simulink model "TetheredUAV_Model"  (R2018a)
settings: Solver=VariableStepAuto  StartTime=0.0  StopTime=200  RelTol=1e-3
undefined symbols (not defined in the file): Discrete, Time, X, Y, Z
libraries: sm_lib x20, simulink x18, nesl_utility x16, commchan3 x5, sharedtransform x1, ctrlSharedLib x1
(part 2 of 2)

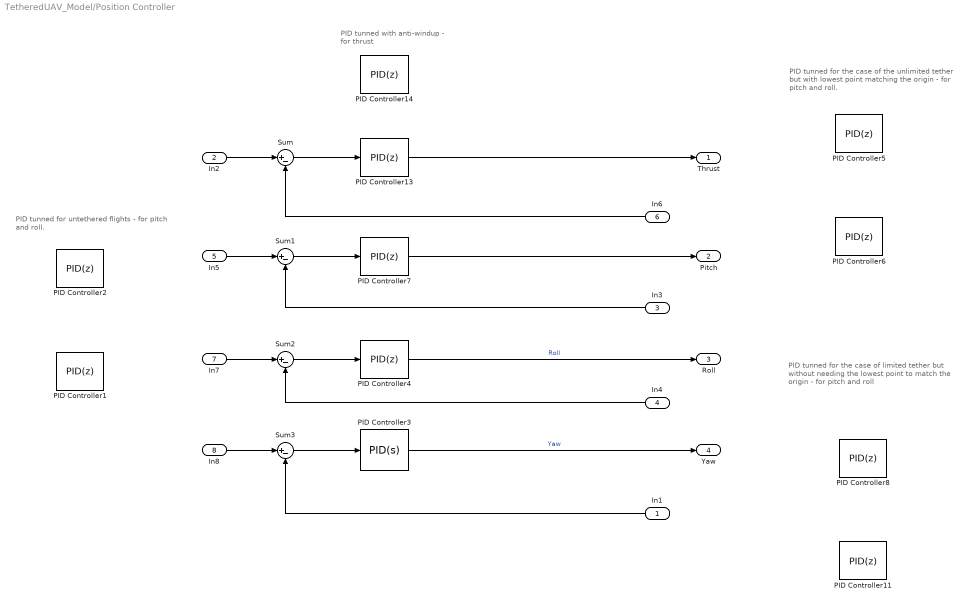
== system TetheredUAV_Model/Position Controller ==
  note: PID tunned with
      | anti-windup - for thrust
  note: PID tunned for the case of the
      | unlimited tether but with lowest
      | point matching the origin - for pitch
      | and roll.
  note: PID tunned for untethered flights -
      | for pitch and roll.
  note: PID tunned for the case of limited
      | tether but without needing the
      | lowest point to match the origin - for
      | pitch and roll
  In1 : Inport
  In2 : Inport  Port=2
  In3 : Inport  Port=3
  In4 : Inport  Port=4
  In5 : Inport  Port=5
  In6 : Inport  Port=6
  In7 : Inport  Port=7
  In8 : Inport  Port=8
  PID Controller1 : simulink/Continuous/PID Controller  Controller=PID  TimeDomain=Discrete-time  SampleTime=0.01  IntegratorMethod=Forward Euler  FilterMethod=Forward Euler  Form=Parallel  UseFilter=off  ControllerParametersSource=internal  P=-0.160436022246273  I=0  D=0  N=44.4052744202431  InitialConditionSource=internal  InitialConditionForIntegrator=0  InitialConditionForFilter=0  ExternalReset=none  LimitOutput=on  UpperSaturationLimit=10  LowerSaturationLimit=-10  LinearizeAsGain=on  AntiWindupMode=none  Kb=1  TrackingMode=off  Kt=1  PParamMin=[]  PParamMax=[]  IParamMin=[]  IParamMax=[]  DParamMin=[]  DParamMax=[]  NParamMin=[]  NParamMax=[]  KbParamMin=[]  KbParamMax=[]  KtParamMin=[]  KtParamMax=[]  POutMin=[]  POutMax=[]  IOutMin=[]  IOutMax=[]  DOutMin=[]  DOutMax=[]  NOutMin=[]  NOutMax=[]  KbOutMin=[]  KbOutMax=[]  KtOutMin=[]  KtOutMax=[]  IntegratorOutMin=[]  IntegratorOutMax=[]  FilterOutMin=[]  FilterOutMax=[]  SumOutMin=[]  SumOutMax=[]  SumI1OutMin=[]  SumI1OutMax=[]  SumI2OutMin=[]  SumI2OutMax=[]  SumI3OutMin=[]  SumI3OutMax=[]  SumDOutMin=[]  SumDOutMax=[]  SaturationOutMin=[]  SaturationOutMax=[]  IntegratorContinuousStateAttributes=''  IntegratorStateMustResolveToSignalObject=off  IntegratorRTWStateStorageClass=Auto  FilterContinuousStateAttributes=''  FilterStateMustResolveToSignalObject=off  FilterRTWStateStorageClass=Auto  DifferentiatorICPrevScaledInput=0  DifferentiatorOutMin=[]  DifferentiatorOutMax=[]  FilterDiffOutCoefMin=[]  FilterDiffOutCoefMax=[]  SumDenOutMin=[]  SumDenOutMax=[]  SumNumOutMin=[]  SumNumOutMax=[]  ReciprocalOutMin=[]  ReciprocalOutMax=[]  DivideOutMin=[]  DivideOutMax=[]  TunerSelectOption=Transfer Function Based (PID Tuner App)
  PID Controller11 : simulink/Continuous/PID Controller  Controller=PID  TimeDomain=Discrete-time  SampleTime=0.01  IntegratorMethod=Forward Euler  FilterMethod=Forward Euler  Form=Parallel  UseFilter=off  ControllerParametersSource=internal  P=-0.1  I=-0.2  D=-15  N=44.4052744202431  InitialConditionSource=internal  InitialConditionForIntegrator=0  InitialConditionForFilter=0  ExternalReset=none  LimitOutput=on  UpperSaturationLimit=10  LowerSaturationLimit=-10  LinearizeAsGain=on  AntiWindupMode=none  Kb=1  TrackingMode=off  Kt=1  PParamMin=[]  PParamMax=[]  IParamMin=[]  IParamMax=[]  DParamMin=[]  DParamMax=[]  NParamMin=[]  NParamMax=[]  KbParamMin=[]  KbParamMax=[]  KtParamMin=[]  KtParamMax=[]  POutMin=[]  POutMax=[]  IOutMin=[]  IOutMax=[]  DOutMin=[]  DOutMax=[]  NOutMin=[]  NOutMax=[]  KbOutMin=[]  KbOutMax=[]  KtOutMin=[]  KtOutMax=[]  IntegratorOutMin=[]  IntegratorOutMax=[]  FilterOutMin=[]  FilterOutMax=[]  SumOutMin=[]  SumOutMax=[]  SumI1OutMin=[]  SumI1OutMax=[]  SumI2OutMin=[]  SumI2OutMax=[]  SumI3OutMin=[]  SumI3OutMax=[]  SumDOutMin=[]  SumDOutMax=[]  SaturationOutMin=[]  SaturationOutMax=[]  IntegratorContinuousStateAttributes=''  IntegratorStateMustResolveToSignalObject=off  IntegratorRTWStateStorageClass=Auto  FilterContinuousStateAttributes=''  FilterStateMustResolveToSignalObject=off  FilterRTWStateStorageClass=Auto  DifferentiatorICPrevScaledInput=0  DifferentiatorOutMin=[]  DifferentiatorOutMax=[]  FilterDiffOutCoefMin=[]  FilterDiffOutCoefMax=[]  SumDenOutMin=[]  SumDenOutMax=[]  SumNumOutMin=[]  SumNumOutMax=[]  ReciprocalOutMin=[]  ReciprocalOutMax=[]  DivideOutMin=[]  DivideOutMax=[]  TunerSelectOption=Transfer Function Based (PID Tuner App)
  PID Controller13 : simulink/Continuous/PID Controller  Controller=PID  TimeDomain=Discrete-time  SampleTime=0.01  IntegratorMethod=Forward Euler  FilterMethod=Forward Euler  Form=Parallel  UseFilter=off  ControllerParametersSource=internal  P=140000  I=7000  D=1000000  N=1  InitialConditionSource=internal  InitialConditionForIntegrator=0  InitialConditionForFilter=0  ExternalReset=none  LimitOutput=on  UpperSaturationLimit=240000  LowerSaturationLimit=40000  LinearizeAsGain=on  AntiWindupMode=none  Kb=1  TrackingMode=off  Kt=1  PParamMin=[]  PParamMax=[]  IParamMin=[]  IParamMax=[]  DParamMin=[]  DParamMax=[]  NParamMin=[]  NParamMax=[]  KbParamMin=[]  KbParamMax=[]  KtParamMin=[]  KtParamMax=[]  POutMin=[]  POutMax=[]  IOutMin=[]  IOutMax=[]  DOutMin=[]  DOutMax=[]  NOutMin=[]  NOutMax=[]  KbOutMin=[]  KbOutMax=[]  KtOutMin=[]  KtOutMax=[]  IntegratorOutMin=[]  IntegratorOutMax=[]  FilterOutMin=[]  FilterOutMax=[]  SumOutMin=[]  SumOutMax=[]  SumI1OutMin=[]  SumI1OutMax=[]  SumI2OutMin=[]  SumI2OutMax=[]  SumI3OutMin=[]  SumI3OutMax=[]  SumDOutMin=[]  SumDOutMax=[]  SaturationOutMin=[]  SaturationOutMax=[]  IntegratorContinuousStateAttributes=''  IntegratorStateMustResolveToSignalObject=off  IntegratorRTWStateStorageClass=Auto  FilterContinuousStateAttributes=''  FilterStateMustResolveToSignalObject=off  FilterRTWStateStorageClass=Auto  DifferentiatorICPrevScaledInput=0  DifferentiatorOutMin=[]  DifferentiatorOutMax=[]  FilterDiffOutCoefMin=[]  FilterDiffOutCoefMax=[]  SumDenOutMin=[]  SumDenOutMax=[]  SumNumOutMin=[]  SumNumOutMax=[]  ReciprocalOutMin=[]  ReciprocalOutMax=[]  DivideOutMin=[]  DivideOutMax=[]  TunerSelectOption=Transfer Function Based (PID Tuner App)
  PID Controller14 : simulink/Continuous/PID Controller  Controller=PID  TimeDomain=Discrete-time  SampleTime=0.01  IntegratorMethod=Forward Euler  FilterMethod=Forward Euler  Form=Parallel  UseFilter=off  ControllerParametersSource=internal  P=140000  I=10000  D=1000000  N=1  InitialConditionSource=internal  InitialConditionForIntegrator=0  InitialConditionForFilter=0  ExternalReset=none  LimitOutput=on  UpperSaturationLimit=240000  LowerSaturationLimit=40000  LinearizeAsGain=on  AntiWindupMode=back-calculation  Kb=1  TrackingMode=off  Kt=1  PParamMin=[]  PParamMax=[]  IParamMin=[]  IParamMax=[]  DParamMin=[]  DParamMax=[]  NParamMin=[]  NParamMax=[]  KbParamMin=[]  KbParamMax=[]  KtParamMin=[]  KtParamMax=[]  POutMin=[]  POutMax=[]  IOutMin=[]  IOutMax=[]  DOutMin=[]  DOutMax=[]  NOutMin=[]  NOutMax=[]  KbOutMin=[]  KbOutMax=[]  KtOutMin=[]  KtOutMax=[]  IntegratorOutMin=[]  IntegratorOutMax=[]  FilterOutMin=[]  FilterOutMax=[]  SumOutMin=[]  SumOutMax=[]  SumI1OutMin=[]  SumI1OutMax=[]  SumI2OutMin=[]  SumI2OutMax=[]  SumI3OutMin=[]  SumI3OutMax=[]  SumDOutMin=[]  SumDOutMax=[]  SaturationOutMin=[]  SaturationOutMax=[]  IntegratorContinuousStateAttributes=''  IntegratorStateMustResolveToSignalObject=off  IntegratorRTWStateStorageClass=Auto  FilterContinuousStateAttributes=''  FilterStateMustResolveToSignalObject=off  FilterRTWStateStorageClass=Auto  DifferentiatorICPrevScaledInput=0  DifferentiatorOutMin=[]  DifferentiatorOutMax=[]  FilterDiffOutCoefMin=[]  FilterDiffOutCoefMax=[]  SumDenOutMin=[]  SumDenOutMax=[]  SumNumOutMin=[]  SumNumOutMax=[]  ReciprocalOutMin=[]  ReciprocalOutMax=[]  DivideOutMin=[]  DivideOutMax=[]  TunerSelectOption=Transfer Function Based (PID Tuner App)
  PID Controller2 : simulink/Continuous/PID Controller  Controller=PID  TimeDomain=Discrete-time  SampleTime=0.01  IntegratorMethod=Forward Euler  FilterMethod=Forward Euler  Form=Parallel  UseFilter=off  ControllerParametersSource=internal  P=0.160436022246273  I=0  D=0  N=44.4052744202431  InitialConditionSource=internal  InitialConditionForIntegrator=0  InitialConditionForFilter=0  ExternalReset=none  LimitOutput=on  UpperSaturationLimit=10  LowerSaturationLimit=-10  LinearizeAsGain=on  AntiWindupMode=none  Kb=1  TrackingMode=off  Kt=1  PParamMin=[]  PParamMax=[]  IParamMin=[]  IParamMax=[]  DParamMin=[]  DParamMax=[]  NParamMin=[]  NParamMax=[]  KbParamMin=[]  KbParamMax=[]  KtParamMin=[]  KtParamMax=[]  POutMin=[]  POutMax=[]  IOutMin=[]  IOutMax=[]  DOutMin=[]  DOutMax=[]  NOutMin=[]  NOutMax=[]  KbOutMin=[]  KbOutMax=[]  KtOutMin=[]  KtOutMax=[]  IntegratorOutMin=[]  IntegratorOutMax=[]  FilterOutMin=[]  FilterOutMax=[]  SumOutMin=[]  SumOutMax=[]  SumI1OutMin=[]  SumI1OutMax=[]  SumI2OutMin=[]  SumI2OutMax=[]  SumI3OutMin=[]  SumI3OutMax=[]  SumDOutMin=[]  SumDOutMax=[]  SaturationOutMin=[]  SaturationOutMax=[]  IntegratorContinuousStateAttributes=''  IntegratorStateMustResolveToSignalObject=off  IntegratorRTWStateStorageClass=Auto  FilterContinuousStateAttributes=''  FilterStateMustResolveToSignalObject=off  FilterRTWStateStorageClass=Auto  DifferentiatorICPrevScaledInput=0  DifferentiatorOutMin=[]  DifferentiatorOutMax=[]  FilterDiffOutCoefMin=[]  FilterDiffOutCoefMax=[]  SumDenOutMin=[]  SumDenOutMax=[]  SumNumOutMin=[]  SumNumOutMax=[]  ReciprocalOutMin=[]  ReciprocalOutMax=[]  DivideOutMin=[]  DivideOutMax=[]  TunerSelectOption=Transfer Function Based (PID Tuner App)
  PID Controller3 : simulink/Continuous/PID Controller  Controller=PID  TimeDomain=Continuous-time  SampleTime=-1  IntegratorMethod=Forward Euler  FilterMethod=Forward Euler  Form=Parallel  UseFilter=on  ControllerParametersSource=internal  P=0  I=0  D=0  N=5.45397025421619  InitialConditionSource=internal  InitialConditionForIntegrator=0  InitialConditionForFilter=0  ExternalReset=none  LimitOutput=off  UpperSaturationLimit=inf  LowerSaturationLimit=-inf  LinearizeAsGain=on  AntiWindupMode=none  Kb=1  TrackingMode=off  Kt=1  PParamMin=[]  PParamMax=[]  IParamMin=[]  IParamMax=[]  DParamMin=[]  DParamMax=[]  NParamMin=[]  NParamMax=[]  KbParamMin=[]  KbParamMax=[]  KtParamMin=[]  KtParamMax=[]  POutMin=[]  POutMax=[]  IOutMin=[]  IOutMax=[]  DOutMin=[]  DOutMax=[]  NOutMin=[]  NOutMax=[]  KbOutMin=[]  KbOutMax=[]  KtOutMin=[]  KtOutMax=[]  IntegratorOutMin=[]  IntegratorOutMax=[]  FilterOutMin=[]  FilterOutMax=[]  SumOutMin=[]  SumOutMax=[]  SumI1OutMin=[]  SumI1OutMax=[]  SumI2OutMin=[]  SumI2OutMax=[]  SumI3OutMin=[]  SumI3OutMax=[]  SumDOutMin=[]  SumDOutMax=[]  SaturationOutMin=[]  SaturationOutMax=[]  IntegratorContinuousStateAttributes=''  IntegratorStateMustResolveToSignalObject=off  IntegratorRTWStateStorageClass=Auto  FilterContinuousStateAttributes=''  FilterStateMustResolveToSignalObject=off  FilterRTWStateStorageClass=Auto  DifferentiatorICPrevScaledInput=0  DifferentiatorOutMin=[]  DifferentiatorOutMax=[]  FilterDiffOutCoefMin=[]  FilterDiffOutCoefMax=[]  SumDenOutMin=[]  SumDenOutMax=[]  SumNumOutMin=[]  SumNumOutMax=[]  ReciprocalOutMin=[]  ReciprocalOutMax=[]  DivideOutMin=[]  DivideOutMax=[]  TunerSelectOption=Transfer Function Based (PID Tuner App)
  PID Controller4 : simulink/Continuous/PID Controller  Controller=PID  TimeDomain=Discrete-time  SampleTime=0.01  IntegratorMethod=Forward Euler  FilterMethod=Forward Euler  Form=Parallel  UseFilter=off  ControllerParametersSource=internal  P=-0.1  I=-0.2  D=-15  N=44.4052744202431  InitialConditionSource=internal  InitialConditionForIntegrator=0  InitialConditionForFilter=0  ExternalReset=none  LimitOutput=on  UpperSaturationLimit=10  LowerSaturationLimit=-10  LinearizeAsGain=on  AntiWindupMode=none  Kb=1  TrackingMode=off  Kt=1  PParamMin=[]  PParamMax=[]  IParamMin=[]  IParamMax=[]  DParamMin=[]  DParamMax=[]  NParamMin=[]  NParamMax=[]  KbParamMin=[]  KbParamMax=[]  KtParamMin=[]  KtParamMax=[]  POutMin=[]  POutMax=[]  IOutMin=[]  IOutMax=[]  DOutMin=[]  DOutMax=[]  NOutMin=[]  NOutMax=[]  KbOutMin=[]  KbOutMax=[]  KtOutMin=[]  KtOutMax=[]  IntegratorOutMin=[]  IntegratorOutMax=[]  FilterOutMin=[]  FilterOutMax=[]  SumOutMin=[]  SumOutMax=[]  SumI1OutMin=[]  SumI1OutMax=[]  SumI2OutMin=[]  SumI2OutMax=[]  SumI3OutMin=[]  SumI3OutMax=[]  SumDOutMin=[]  SumDOutMax=[]  SaturationOutMin=[]  SaturationOutMax=[]  IntegratorContinuousStateAttributes=''  IntegratorStateMustResolveToSignalObject=off  IntegratorRTWStateStorageClass=Auto  FilterContinuousStateAttributes=''  FilterStateMustResolveToSignalObject=off  FilterRTWStateStorageClass=Auto  DifferentiatorICPrevScaledInput=0  DifferentiatorOutMin=[]  DifferentiatorOutMax=[]  FilterDiffOutCoefMin=[]  FilterDiffOutCoefMax=[]  SumDenOutMin=[]  SumDenOutMax=[]  SumNumOutMin=[]  SumNumOutMax=[]  ReciprocalOutMin=[]  ReciprocalOutMax=[]  DivideOutMin=[]  DivideOutMax=[]  TunerSelectOption=Transfer Function Based (PID Tuner App)
  PID Controller5 : simulink/Continuous/PID Controller  Controller=PID  TimeDomain=Discrete-time  SampleTime=0.01  IntegratorMethod=Forward Euler  FilterMethod=Forward Euler  Form=Parallel  UseFilter=off  ControllerParametersSource=internal  P=0.4  I=0.4  D=2  N=44.4052744202431  InitialConditionSource=internal  InitialConditionForIntegrator=0  InitialConditionForFilter=0  ExternalReset=none  LimitOutput=on  UpperSaturationLimit=10  LowerSaturationLimit=-10  LinearizeAsGain=on  AntiWindupMode=none  Kb=1  TrackingMode=off  Kt=1  PParamMin=[]  PParamMax=[]  IParamMin=[]  IParamMax=[]  DParamMin=[]  DParamMax=[]  NParamMin=[]  NParamMax=[]  KbParamMin=[]  KbParamMax=[]  KtParamMin=[]  KtParamMax=[]  POutMin=[]  POutMax=[]  IOutMin=[]  IOutMax=[]  DOutMin=[]  DOutMax=[]  NOutMin=[]  NOutMax=[]  KbOutMin=[]  KbOutMax=[]  KtOutMin=[]  KtOutMax=[]  IntegratorOutMin=[]  IntegratorOutMax=[]  FilterOutMin=[]  FilterOutMax=[]  SumOutMin=[]  SumOutMax=[]  SumI1OutMin=[]  SumI1OutMax=[]  SumI2OutMin=[]  SumI2OutMax=[]  SumI3OutMin=[]  SumI3OutMax=[]  SumDOutMin=[]  SumDOutMax=[]  SaturationOutMin=[]  SaturationOutMax=[]  IntegratorContinuousStateAttributes=''  IntegratorStateMustResolveToSignalObject=off  IntegratorRTWStateStorageClass=Auto  FilterContinuousStateAttributes=''  FilterStateMustResolveToSignalObject=off  FilterRTWStateStorageClass=Auto  DifferentiatorICPrevScaledInput=0  DifferentiatorOutMin=[]  DifferentiatorOutMax=[]  FilterDiffOutCoefMin=[]  FilterDiffOutCoefMax=[]  SumDenOutMin=[]  SumDenOutMax=[]  SumNumOutMin=[]  SumNumOutMax=[]  ReciprocalOutMin=[]  ReciprocalOutMax=[]  DivideOutMin=[]  DivideOutMax=[]  TunerSelectOption=Transfer Function Based (PID Tuner App)
  PID Controller6 : simulink/Continuous/PID Controller  Controller=PID  TimeDomain=Discrete-time  SampleTime=0.01  IntegratorMethod=Forward Euler  FilterMethod=Forward Euler  Form=Parallel  UseFilter=off  ControllerParametersSource=internal  P=-0.4  I=-0.4  D=-2  N=44.4052744202431  InitialConditionSource=internal  InitialConditionForIntegrator=0  InitialConditionForFilter=0  ExternalReset=none  LimitOutput=on  UpperSaturationLimit=10  LowerSaturationLimit=-10  LinearizeAsGain=on  AntiWindupMode=none  Kb=1  TrackingMode=off  Kt=1  PParamMin=[]  PParamMax=[]  IParamMin=[]  IParamMax=[]  DParamMin=[]  DParamMax=[]  NParamMin=[]  NParamMax=[]  KbParamMin=[]  KbParamMax=[]  KtParamMin=[]  KtParamMax=[]  POutMin=[]  POutMax=[]  IOutMin=[]  IOutMax=[]  DOutMin=[]  DOutMax=[]  NOutMin=[]  NOutMax=[]  KbOutMin=[]  KbOutMax=[]  KtOutMin=[]  KtOutMax=[]  IntegratorOutMin=[]  IntegratorOutMax=[]  FilterOutMin=[]  FilterOutMax=[]  SumOutMin=[]  SumOutMax=[]  SumI1OutMin=[]  SumI1OutMax=[]  SumI2OutMin=[]  SumI2OutMax=[]  SumI3OutMin=[]  SumI3OutMax=[]  SumDOutMin=[]  SumDOutMax=[]  SaturationOutMin=[]  SaturationOutMax=[]  IntegratorContinuousStateAttributes=''  IntegratorStateMustResolveToSignalObject=off  IntegratorRTWStateStorageClass=Auto  FilterContinuousStateAttributes=''  FilterStateMustResolveToSignalObject=off  FilterRTWStateStorageClass=Auto  DifferentiatorICPrevScaledInput=0  DifferentiatorOutMin=[]  DifferentiatorOutMax=[]  FilterDiffOutCoefMin=[]  FilterDiffOutCoefMax=[]  SumDenOutMin=[]  SumDenOutMax=[]  SumNumOutMin=[]  SumNumOutMax=[]  ReciprocalOutMin=[]  ReciprocalOutMax=[]  DivideOutMin=[]  DivideOutMax=[]  TunerSelectOption=Transfer Function Based (PID Tuner App)
  PID Controller7 : simulink/Continuous/PID Controller  Controller=PID  TimeDomain=Discrete-time  SampleTime=0.01  IntegratorMethod=Forward Euler  FilterMethod=Forward Euler  Form=Parallel  UseFilter=off  ControllerParametersSource=internal  P=0.1  I=0.2  D=15  N=44.4052744202431  InitialConditionSource=internal  InitialConditionForIntegrator=0  InitialConditionForFilter=0  ExternalReset=none  LimitOutput=on  UpperSaturationLimit=10  LowerSaturationLimit=-10  LinearizeAsGain=on  AntiWindupMode=none  Kb=1  TrackingMode=off  Kt=1  PParamMin=[]  PParamMax=[]  IParamMin=[]  IParamMax=[]  DParamMin=[]  DParamMax=[]  NParamMin=[]  NParamMax=[]  KbParamMin=[]  KbParamMax=[]  KtParamMin=[]  KtParamMax=[]  POutMin=[]  POutMax=[]  IOutMin=[]  IOutMax=[]  DOutMin=[]  DOutMax=[]  NOutMin=[]  NOutMax=[]  KbOutMin=[]  KbOutMax=[]  KtOutMin=[]  KtOutMax=[]  IntegratorOutMin=[]  IntegratorOutMax=[]  FilterOutMin=[]  FilterOutMax=[]  SumOutMin=[]  SumOutMax=[]  SumI1OutMin=[]  SumI1OutMax=[]  SumI2OutMin=[]  SumI2OutMax=[]  SumI3OutMin=[]  SumI3OutMax=[]  SumDOutMin=[]  SumDOutMax=[]  SaturationOutMin=[]  SaturationOutMax=[]  IntegratorContinuousStateAttributes=''  IntegratorStateMustResolveToSignalObject=off  IntegratorRTWStateStorageClass=Auto  FilterContinuousStateAttributes=''  FilterStateMustResolveToSignalObject=off  FilterRTWStateStorageClass=Auto  DifferentiatorICPrevScaledInput=0  DifferentiatorOutMin=[]  DifferentiatorOutMax=[]  FilterDiffOutCoefMin=[]  FilterDiffOutCoefMax=[]  SumDenOutMin=[]  SumDenOutMax=[]  SumNumOutMin=[]  SumNumOutMax=[]  ReciprocalOutMin=[]  ReciprocalOutMax=[]  DivideOutMin=[]  DivideOutMax=[]  TunerSelectOption=Transfer Function Based (PID Tuner App)
  PID Controller8 : simulink/Continuous/PID Controller  Controller=PID  TimeDomain=Discrete-time  SampleTime=0.01  IntegratorMethod=Forward Euler  FilterMethod=Forward Euler  Form=Parallel  UseFilter=off  ControllerParametersSource=internal  P=0.1  I=0.2  D=15  N=44.4052744202431  InitialConditionSource=internal  InitialConditionForIntegrator=0  InitialConditionForFilter=0  ExternalReset=none  LimitOutput=on  UpperSaturationLimit=10  LowerSaturationLimit=-10  LinearizeAsGain=on  AntiWindupMode=none  Kb=1  TrackingMode=off  Kt=1  PParamMin=[]  PParamMax=[]  IParamMin=[]  IParamMax=[]  DParamMin=[]  DParamMax=[]  NParamMin=[]  NParamMax=[]  KbParamMin=[]  KbParamMax=[]  KtParamMin=[]  KtParamMax=[]  POutMin=[]  POutMax=[]  IOutMin=[]  IOutMax=[]  DOutMin=[]  DOutMax=[]  NOutMin=[]  NOutMax=[]  KbOutMin=[]  KbOutMax=[]  KtOutMin=[]  KtOutMax=[]  IntegratorOutMin=[]  IntegratorOutMax=[]  FilterOutMin=[]  FilterOutMax=[]  SumOutMin=[]  SumOutMax=[]  SumI1OutMin=[]  SumI1OutMax=[]  SumI2OutMin=[]  SumI2OutMax=[]  SumI3OutMin=[]  SumI3OutMax=[]  SumDOutMin=[]  SumDOutMax=[]  SaturationOutMin=[]  SaturationOutMax=[]  IntegratorContinuousStateAttributes=''  IntegratorStateMustResolveToSignalObject=off  IntegratorRTWStateStorageClass=Auto  FilterContinuousStateAttributes=''  FilterStateMustResolveToSignalObject=off  FilterRTWStateStorageClass=Auto  DifferentiatorICPrevScaledInput=0  DifferentiatorOutMin=[]  DifferentiatorOutMax=[]  FilterDiffOutCoefMin=[]  FilterDiffOutCoefMax=[]  SumDenOutMin=[]  SumDenOutMax=[]  SumNumOutMin=[]  SumNumOutMax=[]  ReciprocalOutMin=[]  ReciprocalOutMax=[]  DivideOutMin=[]  DivideOutMax=[]  TunerSelectOption=Transfer Function Based (PID Tuner App)
  Sum{,1..3} (4 alike) : Sum  Inputs=|+-
  Thrust : Outport
  Pitch : Outport  Port=2
  Roll : Outport  Port=3
  Yaw : Outport  Port=4
  wires:
  Sum3/1 -> PID Controller3/1
  In1/1 -> Sum3/2
  PID Controller4/1 -> Roll/1  "Roll"
  In8/1 -> Sum3/1
  In2/1 -> Sum/1
  Sum2/1 -> PID Controller4/1
  In6/1 -> Sum/2
  PID Controller3/1 -> Yaw/1  "Yaw"
  In4/1 -> Sum2/2
  PID Controller7/1 -> Pitch/1
  Sum1/1 -> PID Controller7/1
  Sum/1 -> PID Controller13/1
  PID Controller13/1 -> Thrust/1
  In3/1 -> Sum1/2
  In5/1 -> Sum1/1
  In7/1 -> Sum2/1

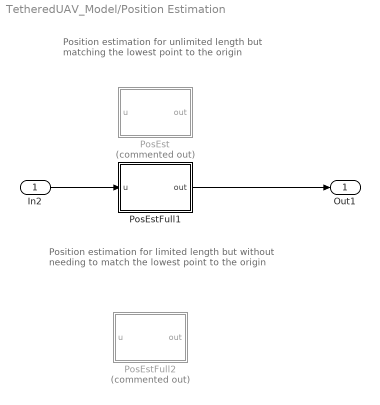
== system TetheredUAV_Model/Position Estimation ==
  note: Position estimation for limited length
      | but without needing to match the
      | lowest point to the origin
  note: Position estimation for unlimited
      | length but matching the lowest point
      | to the origin
  In2 : Inport
  PosEst : MATLAB Function  Commented=on  TreatAsAtomicUnit=on
  PosEstFull1 : MATLAB Function  TreatAsAtomicUnit=on
  PosEstFull2 : MATLAB Function  Commented=on  TreatAsAtomicUnit=on
  Out1 : Outport
  wires:
  PosEstFull1/1(out) -> Out1/1
  In2/1 -> PosEstFull1/1(u)

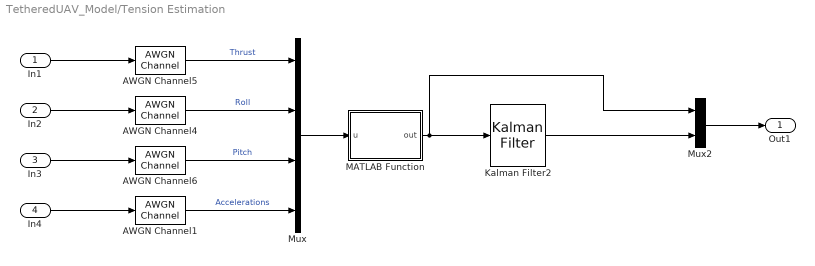
== system TetheredUAV_Model/Tension Estimation ==
  In1 : Inport
  In2 : Inport  Port=2
  In3 : Inport  Port=3
  In4 : Inport  Port=4
  AWGN Channel1 : commchan3/AWGN Channel  InputProcessing=Columns as channels (frame based)  seed=67  noiseMode="Signal to noise ratio  (SNR)"  EbNodB=10  EsNodB=10  SNRdB=30  bitsPerSym=1  Ps=1  Tsym=1  variance=1
  AWGN Channel4 : commchan3/AWGN Channel  InputProcessing=Columns as channels (frame based)  seed=67  noiseMode="Signal to noise ratio  (SNR)"  EbNodB=10  EsNodB=10  SNRdB=40  bitsPerSym=1  Ps=1  Tsym=1  variance=1
  AWGN Channel5 : commchan3/AWGN Channel  InputProcessing=Columns as channels (frame based)  seed=67  noiseMode="Signal to noise ratio  (SNR)"  EbNodB=10  EsNodB=10  SNRdB=40  bitsPerSym=1  Ps=1  Tsym=1  variance=1
  AWGN Channel6 : commchan3/AWGN Channel  InputProcessing=Columns as channels (frame based)  seed=67  noiseMode="Signal to noise ratio  (SNR)"  EbNodB=10  EsNodB=10  SNRdB=40  bitsPerSym=1  Ps=1  Tsym=1  variance=1
  Kalman Filter2 : ctrlSharedLib/Kalman Filter  TimeDomain=Discrete-Time  UseCurrentEstimator=on  ModelSource=Individual A, B, C, D matrices  ModelSourceVariable=ss(0.95,1,1,0,1)  A=eye(3)  B=0  C=eye(3)  D=0  NumberOfStates=1  NumberOfInputs=1  NumberOfOutputs=1  InitialEstimateSource=Dialog  X0=0  P0=10  UseK=off  UseGH=off  NumberOfProcessNoiseInputs=1  G=1  TimeInvariantG=on  H=0  TimeInvariantH=on  Q=diag([1 1 1])  TimeInvariantQ=on  R=100000*eye(3)  TimeInvariantR=on  N=0  TimeInvariantN=on  AddInputPort=off  AddEnablePort=off  OutputEstimatedY=off  OutputP=off  Ts=-1
      settings: SourceProductBaseCode=CT
  MATLAB Function : MATLAB Function  TreatAsAtomicUnit=on
  Mux : Mux
  Mux2 : Mux  Inputs=2
  Out1 : Outport
  wires:
  Mux/1 -> MATLAB Function/1(u)
  Mux2/1 -> Out1/1
  MATLAB Function/1(out) -> Kalman Filter2/1, Mux2/1
  Kalman Filter2/1 -> Mux2/2
  In3/1 -> AWGN Channel6/1
  In2/1 -> AWGN Channel4/1
  In4/1 -> AWGN Channel1/1
  In1/1 -> AWGN Channel5/1
  AWGN Channel4/1 -> Mux/2  "Roll"
  AWGN Channel6/1 -> Mux/3  "Pitch"
  AWGN Channel1/1 -> Mux/4  "Accelerations"
  AWGN Channel5/1 -> Mux/1  "Thrust"

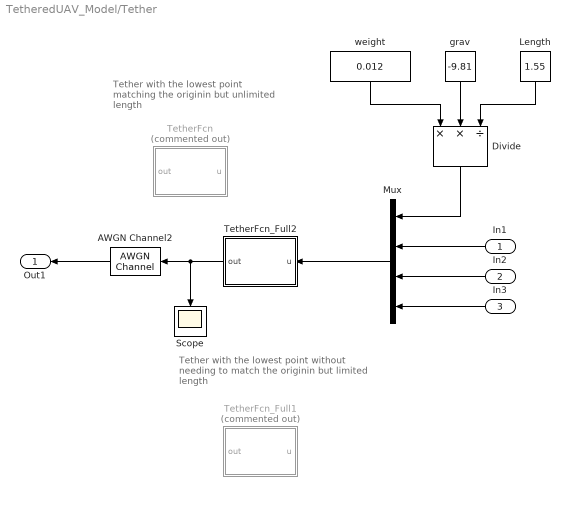
== system TetheredUAV_Model/Tether ==
  note: Tether with the lowest point
      | without needing to match the
      | originin but limited length
  note: Tether with the lowest point
      | matching the originin but
      | unlimited length
  In1 : Inport
  In2 : Inport  Port=2
  In3 : Inport  Port=3
  AWGN Channel2 : commchan3/AWGN Channel  InputProcessing=Columns as channels (frame based)  seed=67  noiseMode="Signal to noise ratio  (SNR)"  EbNodB=10  EsNodB=10  SNRdB=70  bitsPerSym=1  Ps=1  Tsym=1  variance=1
  Divide : Product  Inputs=**/
  Length : Constant  Value=1.55
  Mux : Mux
  Scope : Scope
  TetherFcn : MATLAB Function  Commented=on  TreatAsAtomicUnit=on
  TetherFcn_Full1 : MATLAB Function  Commented=on  TreatAsAtomicUnit=on
  TetherFcn_Full2 : MATLAB Function  TreatAsAtomicUnit=on
  grav : Constant  Value=-9.81
  weight : Constant  Value=0.012
  Out1 : Outport
  wires:
  TetherFcn_Full2/1(out) -> AWGN Channel2/1, Scope/1
  weight/1 -> Divide/1
  Length/1 -> Divide/3
  Divide/1 -> Mux/1
  In1/1 -> Mux/2
  In2/1 -> Mux/3
  In3/1 -> Mux/4
  Mux/1 -> TetherFcn_Full2/1(u)
  grav/1 -> Divide/2
  AWGN Channel2/1 -> Out1/1

== matlab function TetheredUAV_Model/Position Estimation/PosEstFull2 ==
  data: u input; out output
function out = fcn(u)
w=0.012/1.55*9.81;
s_tot=1.55;
% ---- Before Kalman - Raw observations
Tx=-u(4);
Ty=-u(5);
Tz=-u(6);
zi=0.754;
ri=0;

%Obtain the "a" and "s" parameters from the tension
T0=sqrt(Tx^2+Ty^2);
a=T0/w;
s=Tz/w;

%Obtain the r0, r(radial distance), C and z(altitude)
r0=a*asinh((s_tot-s)/a);
r=r0+a*asinh(s/a);
C=zi-a*cosh((ri-r0)/a);
z=a*cosh((r-r0)/a)+C;

%Decomposition of the r
teta=atan2(Ty,Tx);
y=r*sin(teta);
x=r*cos(teta);

out = [x,y,z];

== matlab function TetheredUAV_Model/Motor Controller/MATLAB Function1 ==
  data: u input; y output
function y = fcn(u)
f=u(1);
t1=u(2);
t2=u(3);
t3=u(4);

d=sqrt(2)/2*(0.5-0.025);
c=1;

vec=[f,t1,t2,t3]';
Matrix=[1,1,1,1;0,d,0,-d;-d,0,d,0;-c,c,-c,c];

y=(Matrix)\vec;
y=2.130925*10^(-11)*y.^2+1.032633*10^(-6)*y+5.484560*10^-4;

== matlab function TetheredUAV_Model/Motor Controller/MATLAB Function2 ==
  data: u input; y output
function y = fcn(u)
f=u(1);
t1=u(2);
t2=u(3);
t3=u(4);

d=sqrt(2)/2*(0.5-0.025);
c=1;

vec=[f,t1,t2,t3]';
%Matrix=[1,1,1,1;0,d,0,-d;-d,0,d,0;-c,c,-c,c];
Matrix=[1,1,1,1;-d,d,d,-d;-d,-d,d,d;-c,c,-c,c];

y=(Matrix)\vec;
y=2.130925*10^(-11)*y.^2+1.032633*10^(-6)*y+5.484560*10^-4;

== matlab function TetheredUAV_Model/Tether/TetherFcn_Full1 ==
  data: u input; out output
function out = fcn(u)
w=u(1); %PESO (não massa) por unidade de comprimento
x=u(2);
y=u(3);
z=u(4);
s_tot=1.55;
teta=atan2(y,x);

r=sqrt(x^2+y^2);
ri=0;
zi=0.754;

deltaR=abs(r-ri)/2;
deltaZ=z-zi;
r_av=abs(r+ri)/2;

alfa=sinh(atanh(deltaZ/s_tot));

% Aproximação de Taylor/Maclaurin ordem 5
a=deltaZ/(2*alfa)-deltaR;
b=-deltaR^3/factorial(3);
c=-deltaR^5/factorial(5);

x1=(-b+sqrt(b^2-4*a*c))/(2*a);
a=sqrt(x1); 
%Está 0.1 em vez de 0.01 por causa do deltaZ ser 0. Para valores de r muito
%pequeno o 'a' da corda é ainda mais pequeno (bastante) pelo que a outra
%solução para ter um 'a' com enough precision seria diminuir o erro em
%muito do while. Optei por esta que é mais pratica e 10cm tmb nao é assim
%tanto.
if(r>0.1)
    % Método de Newton-Raphson para calcular o 'a'
    f=inf;
    i=0;
    A=atanh(deltaZ/s_tot);
    while(abs(f)>0.01)
        f=deltaZ-2*a*sinh(atanh(deltaZ/s_tot))*sinh(deltaR/a);
        df=2*sinh(A)*(deltaR/a*cosh(deltaR/a)-sinh(deltaR/a));
        a=a-f/df;
        i=i+1;
    end
    x0_f=r_av-a*atanh(deltaZ/s_tot);

    T0=a*w;
    s=a*sinh((r-x0_f)/a);
else
    s=(s_tot+z-zi)/2;
    T0=0;
end
Tz=s*w;

Tx=cos(teta)*T0;
Ty=sin(teta)*T0;
out=[Tx, Ty, Tz];

== matlab function TetheredUAV_Model/Motor Controller/MATLAB Function3 ==
  data: u input; y output
function y = fcn(u)
f=u(1);
t1=u(2);
t2=u(3);
t3=u(4);

d=sqrt(2)/2*(0.5-0.025);
c=1;

vec=[f,t1,t2,t3]';
%Matrix=[1,1,1,1;0,d,0,-d;-d,0,d,0;-c,c,-c,c];
Matrix=[1,1,1,1;-d,-d,d,d;-d,d,d,-d;-c,c,-c,c];

y=(Matrix)\vec;
y=2.130925*10^(-11)*y.^2+1.032633*10^(-6)*y+5.484560*10^-4;

== matlab function TetheredUAV_Model/Tension Estimation/MATLAB Function ==
  settings: updateMethod=DISCRETE
  data: u input; out output
function out = fcn(u)
%---Inputs ---
Fp=u(1);
roll=u(2);
pitch=u(3);
accX=u(4);
accY=u(5);
accZ=u(6);

yaw=0;
mass=0.03;

%----Rotation matrix indices----
a=cos(yaw)*cos(pitch);
b=-sin(yaw)*cos(roll)+cos(yaw)*sin(pitch)*sin(roll);
c=sin(yaw)*sin(roll)+cos(yaw)*sin(pitch)*cos(roll);
 
d=sin(yaw)*cos(pitch);
e=cos(yaw)*cos(roll)+sin(yaw)*sin(pitch)*sin(roll);
f=-cos(yaw)*sin(roll)+sin(yaw)*sin(pitch)*cos(roll);
 
g=-sin(pitch);
h=cos(pitch)*sin(roll);
i=cos(pitch)*cos(roll);

%----Positive tension when pulling in the same direction of the axes!----
Tx=mass*accX-c*Fp;
Ty=mass*accY-f*Fp;
Tz=mass*(accZ+9.81)-i*Fp;


out=[Tx, Ty, Tz];

== matlab function TetheredUAV_Model/Position Estimation/PosEstFull1 ==
  data: u input; out output
function out = fcn(u)
w=0.012/1.55*9.81;
s_tot=1.55;
% ---- Before Kalman - Raw observations
Tx=-u(4);
Ty=-u(5);
Tz=-u(6);
zi=0.754;
ri=0;

%valores obtidos através das tensões são o a e o x0
T0=sqrt(Tx^2+Ty^2);
a=T0/w;
s=Tz/w;

%Descobir o r atual, o r0 e o C
r0=a*asinh((s_tot-s)/a);
r=r0+a*asinh(s/a);
C=zi-a*cosh((ri-r0)/a);
z=a*cosh((r-r0)/a)+C;
teta=atan2(Ty,Tx);
y=r*sin(teta);
x=r*cos(teta);

% ---- After Kalman - Filtered observations
Tx2=u(4);
Ty2=u(5);
Tz2=u(6);

T02=sqrt(Tx2^2+Ty2^2);
a2=T02/w;
s2=Tz2/w;
r2=asinh(s2/a2)*a2;
z2=a2*cosh(r2/a2)-a2;
teta2=atan2(Ty2,Tx2);
y2=r2*sin(teta2);
x2=r2*cos(teta2);


out = [x,y,z];

== matlab function TetheredUAV_Model/Euler2angles1 ==
  data: u input; y output
function y = fcn(u)
roll=u(2);
pitch=u(1);

y=zeros(1,2);
y(1)=roll*180/pi;
y(2)=pitch*180/pi;

== matlab function TetheredUAV_Model/Motor Controller/MATLAB Function4 ==
  data: u input; out output
function out = fcn(u)
f=u(1);
t1=u(2);
t2=u(3);
t3=u(4);

d=(0.5-0.025);
c=1;

vec=[f,t1,t2,t3]';
Matrix=[1,1,1,1;0,d,0,-d;-d,0,d,0;-c,c,-c,c];
Matrix2=[1,1,1,1;-d,d,d,-d;-d,-d,d,d;-c,c,-c,c];
y2=(Matrix2)\vec;
y=(Matrix)\vec;
y=2.130925*10^(-11)*y.^2+1.032633*10^(-6)*y+5.484560*10^-4;
y2=2.130925*10^(-11)*y2.^2+1.032633*10^(-6)*y2+5.484560*10^-4;
out=[y];

== matlab function TetheredUAV_Model/Plant/MATLAB Function1 ==
  data: u input; y output
function y = fcn(u)
    y=-(1000*u(1)+100*u(2));
end

== matlab function TetheredUAV_Model/Tether/TetherFcn_Full2 ==
  data: u input; out output
function out = fcn(u)
w=u(1); %PESO (não massa) por unidade de comprimento
x=u(2);
y=u(3);
z=u(4);
s_tot=1.55;
teta=atan2(y,x);

r=sqrt(x^2+y^2);
ri=0;
zi=0.754;

deltaR=abs(r-ri)/2;
deltaZ=z-zi;
r_av=abs(r+ri)/2;

alfa=sinh(atanh(deltaZ/s_tot));

% Aproximação de Taylor/Maclaurin ordem 5
a=deltaZ/(2*alfa)-deltaR;
b=-deltaR^3/factorial(3);
c=-deltaR^5/factorial(5);

x1=(-b+sqrt(b^2-4*a*c))/(2*a);
a=sqrt(x1); 
%Está 0.1 em vez de 0.01 por causa do deltaZ ser 0. Para valores de r muito
%pequeno o 'a' da corda é ainda mais pequeno (bastante) pelo que a outra
%solução para ter um 'a' com enough precision seria diminuir o erro em
%muito do while. Optei por esta que é mais pratica e 10cm tmb nao é assim
%tanto.
if(r>0.1)
    % Método de Newton-Raphson para calcular o 'a'
    f=inf;
    i=0;
    A=atanh(deltaZ/s_tot);
    while(abs(f)>0.01)
        f=deltaZ-2*a*sinh(atanh(deltaZ/s_tot))*sinh(deltaR/a);
        df=2*sinh(A)*(deltaR/a*cosh(deltaR/a)-sinh(deltaR/a));
        a=a-f/df;
        i=i+1;
    end
    x0_f=r_av-a*atanh(deltaZ/s_tot);

    T0=a*w;
    s=a*sinh((r-x0_f)/a);
else
    s=(s_tot+z-zi)/2;
    T0=0;
end
Tz=s*w;

Tx=cos(teta)*T0;
Ty=sin(teta)*T0;
out=[Tx, Ty, Tz];

== matlab function TetheredUAV_Model/Tether/TetherFcn ==
  data: u input; out output
function out = fcn(u)
w=u(1); %PESO (não massa) por unidade de comprimento
x=u(2);
y=u(3);
z=u(4);

r=sqrt(x^2+y^2);

count=0;
if(r>=0.05)
    %Função para encontrar a melhor estimativa
    a=z; b=-r^2; d=-r^4/factorial(4);

    p=-b^2/(3*a^2);
    q=(2*b^3+27*a^2*d)/(27*a^3);

    aux=(-q/2+sqrt(q^2/4+p^3/27))^(1/3)+(-q/2-sqrt(q^2/4+p^3/27))^(1/3);
    %----------

    c=aux; %Este primeiro valor de 'c' corresponde à estimativa
    erro=inf;
    while(erro>0.01)
        f=z-(c*cosh(r/c)-c);
        df=r/c*sinh(r/c)-cosh(r/c)+1;

        c=c-f/df;
        erro=abs(f);
        count=count+1;
    end

    s=c*sinh(r/c);
    T0=c*w;
    teta=atan2(y,x);
    Tx=cos(teta)*T0;
    Ty=sin(teta)*T0;
else
    s=z;
    T0=0;
    Tx=0;
    Ty=0;
    teta=-1;
end

T_vert=w*s;

out=[Tx,Ty,T_vert];

== matlab function TetheredUAV_Model/Position Estimation/PosEst ==
  data: u input; out output
function out = fcn(u)
w=0.012/1.55*9.81;

%Before Kalman - Raw observations
Tx=u(1);
Ty=u(2);
Tz=u(3);

T0=sqrt(Tx^2+Ty^2);
a=T0/w;
s=Tz/w;
r=asinh(s/a)*a;
z=a*cosh(r/a)-a;
teta=atan2(Ty,Tx);
y=r*sin(teta);
x=r*cos(teta);

%After Kalman - Filtered observations
Tx2=u(4);
Ty2=u(5);
Tz2=u(6);

T02=sqrt(Tx2^2+Ty2^2);
a2=T02/w;
s2=Tz2/w;
r2=asinh(s2/a2)*a2;
z2=a2*cosh(r2/a2)-a2;
teta2=atan2(Ty2,Tx2);
y2=r2*sin(teta2);
x2=r2*cos(teta2);


out = [x2,y2,z2];
